simulink model "constraints_comparison_A_4D_v2"  (R2017b)
settings: Solver=ode4  StartTime=0.0  StopTime=10  FixedStep=0.0001  RelTol=1e-3  EnableMultiTasking=on
InitFcn:
  | clear
  | clc
values from neighbouring files (symbols this model uses):
  dail = aircraft_response.Data(:,9)    [dutch_roll_responses_test_plot.m]    (also in short_period_phugoid_responses_test.m)
  dele = aircraft_response.Data(:,10)    [dutch_roll_responses_test_plot.m]    (also in short_period_phugoid_responses_test.m)
  drud = aircraft_response.Data(:,11)    [dutch_roll_responses_test_plot.m]    (also in short_period_phugoid_responses_test.m)
undefined symbols (not defined in the file or in its folder): acm_aero_model, acm_T_N, breakpoints1, Cm0, Cmde, Cmq, de, Fr_mp_1, Fr_mp_2, Fr_rp_1, Fr_rp_2, ini_acm_de_deg, ini_acm_p_deg_per_s, ini_acm_phi_deg, ini_acm_psi_deg, ini_acm_q_deg_per_s, ini_acm_r_deg_per_s, ini_acm_theta_deg, ini_cmp_de_deg, ini_rig_p_deg_per_s, ini_rig_phi_deg, ini_rig_psi_deg, ini_rig_q_deg_per_s, ini_rig_r_deg_per_s, ini_rig_theta_deg, K1_svo_acm, K1_svo_cmp, K2_svo_acm, K2_svo_cmp, La, Ma, max_defl_sat_acm, max_defl_sat_cmp, max_rate_sat, max_rate_sat_acm, max_rate_sat_cmp, Na, sigbuilder_block, simstop, windspeed, Xa, Ya, Za
libraries: aerolibconvert2 x117, simulink x35, sharedtransform x19, vrlib x2
(part 3 of 5)

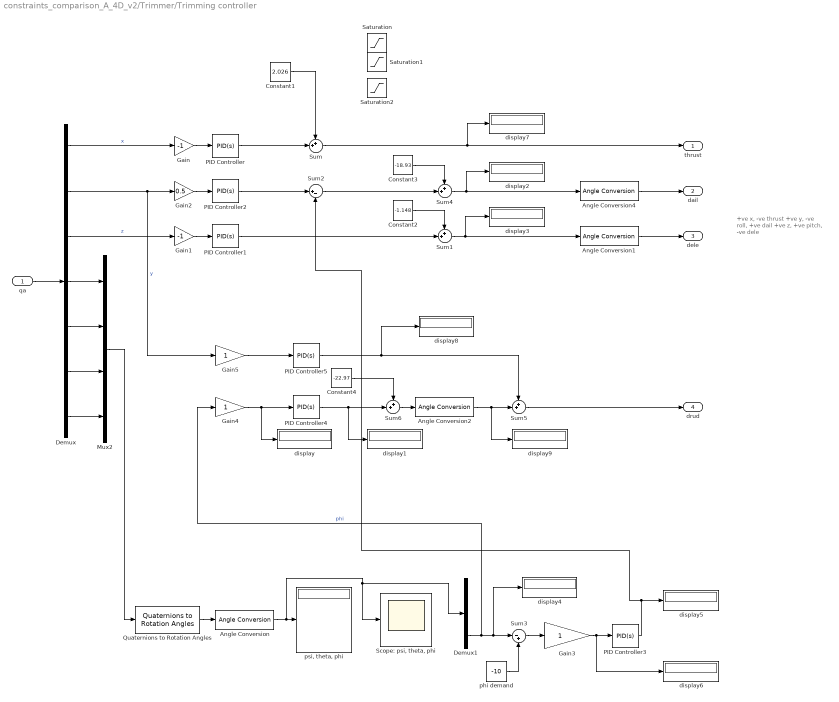
== system constraints_comparison_A_4D_v2/Trimmer/Trimming controller ==
  note: +ve x, -ve thrust
      |
      | +ve y, -ve roll, +ve dail
      |
      | +ve z, +ve pitch, -ve dele
  qa : Inport
  Angle Conversion : aerolibconvert2/Angle Conversion  IU=rad  OU=deg
  Angle Conversion1 : aerolibconvert2/Angle Conversion  IU=deg  OU=rad
  Angle Conversion2 : aerolibconvert2/Angle Conversion  IU=deg  OU=rad
  Angle Conversion4 : aerolibconvert2/Angle Conversion  IU=deg  OU=rad
  Constant1 : Constant  Value=2.026
  Constant2 : Constant  Value=-1.148
  Constant3 : Constant  Value=-18.93
  Constant4 : Constant  Value=-22.97
  Demux : Demux  Outputs=7
  Demux1 : Demux  Outputs=3
  Gain : Gain  Gain=-1
  Gain1 : Gain  Gain=-1
  Gain2 : Gain  Gain=0.5
  Gain3 : Gain
  Gain4 : Gain
  Gain5 : Gain
  Mux2 : Mux
  PID Controller : simulink/Continuous/PID Controller  Controller=PID  TimeDomain=Continuous-time  SampleTime=-1  IntegratorMethod=Forward Euler  FilterMethod=Forward Euler  Form=Parallel  UseFilter=on  ControllerParametersSource=internal  P=2  I=0.5  D=1  N=100  InitialConditionSource=internal  InitialConditionForIntegrator=0  InitialConditionForFilter=0  ExternalReset=none  LimitOutput=off  UpperSaturationLimit=inf  LowerSaturationLimit=-inf  LinearizeAsGain=on  AntiWindupMode=none  Kb=1  TrackingMode=off  Kt=1  PParamMin=[]  PParamMax=[]  IParamMin=[]  IParamMax=[]  DParamMin=[]  DParamMax=[]  NParamMin=[]  NParamMax=[]  KbParamMin=[]  KbParamMax=[]  KtParamMin=[]  KtParamMax=[]  POutMin=[]  POutMax=[]  IOutMin=[]  IOutMax=[]  DOutMin=[]  DOutMax=[]  NOutMin=[]  NOutMax=[]  KbOutMin=[]  KbOutMax=[]  KtOutMin=[]  KtOutMax=[]  IntegratorOutMin=[]  IntegratorOutMax=[]  FilterOutMin=[]  FilterOutMax=[]  SumOutMin=[]  SumOutMax=[]  SumI1OutMin=[]  SumI1OutMax=[]  SumI2OutMin=[]  SumI2OutMax=[]  SumI3OutMin=[]  SumI3OutMax=[]  SumDOutMin=[]  SumDOutMax=[]  SaturationOutMin=[]  SaturationOutMax=[]  IntegratorContinuousStateAttributes=''  IntegratorStateMustResolveToSignalObject=off  IntegratorRTWStateStorageClass=Auto  FilterContinuousStateAttributes=''  FilterStateMustResolveToSignalObject=off  FilterRTWStateStorageClass=Auto  DifferentiatorICPrevScaledInput=0  DifferentiatorOutMin=[]  DifferentiatorOutMax=[]  InitialConditionSetting=State (most efficient)  FilterDiffOutCoefMin=[]  FilterDiffOutCoefMax=[]  SumDenOutMin=[]  SumDenOutMax=[]  SumNumOutMin=[]  SumNumOutMax=[]  ReciprocalOutMin=[]  ReciprocalOutMax=[]  DivideOutMin=[]  DivideOutMax=[]  TunerSelectOption=Transfer Function Based (PID Tuner App)
  PID Controller1 : simulink/Continuous/PID Controller  Controller=PID  TimeDomain=Continuous-time  SampleTime=-1  IntegratorMethod=Forward Euler  FilterMethod=Forward Euler  Form=Parallel  UseFilter=on  ControllerParametersSource=internal  P=2  I=0.5  D=1  N=100  InitialConditionSource=internal  InitialConditionForIntegrator=0  InitialConditionForFilter=0  ExternalReset=none  LimitOutput=off  UpperSaturationLimit=inf  LowerSaturationLimit=-inf  LinearizeAsGain=on  AntiWindupMode=none  Kb=1  TrackingMode=off  Kt=1  PParamMin=[]  PParamMax=[]  IParamMin=[]  IParamMax=[]  DParamMin=[]  DParamMax=[]  NParamMin=[]  NParamMax=[]  KbParamMin=[]  KbParamMax=[]  KtParamMin=[]  KtParamMax=[]  POutMin=[]  POutMax=[]  IOutMin=[]  IOutMax=[]  DOutMin=[]  DOutMax=[]  NOutMin=[]  NOutMax=[]  KbOutMin=[]  KbOutMax=[]  KtOutMin=[]  KtOutMax=[]  IntegratorOutMin=[]  IntegratorOutMax=[]  FilterOutMin=[]  FilterOutMax=[]  SumOutMin=[]  SumOutMax=[]  SumI1OutMin=[]  SumI1OutMax=[]  SumI2OutMin=[]  SumI2OutMax=[]  SumI3OutMin=[]  SumI3OutMax=[]  SumDOutMin=[]  SumDOutMax=[]  SaturationOutMin=[]  SaturationOutMax=[]  IntegratorContinuousStateAttributes=''  IntegratorStateMustResolveToSignalObject=off  IntegratorRTWStateStorageClass=Auto  FilterContinuousStateAttributes=''  FilterStateMustResolveToSignalObject=off  FilterRTWStateStorageClass=Auto  DifferentiatorICPrevScaledInput=0  DifferentiatorOutMin=[]  DifferentiatorOutMax=[]  InitialConditionSetting=State (most efficient)  FilterDiffOutCoefMin=[]  FilterDiffOutCoefMax=[]  SumDenOutMin=[]  SumDenOutMax=[]  SumNumOutMin=[]  SumNumOutMax=[]  ReciprocalOutMin=[]  ReciprocalOutMax=[]  DivideOutMin=[]  DivideOutMax=[]  TunerSelectOption=Transfer Function Based (PID Tuner App)
  PID Controller2 : simulink/Continuous/PID Controller  Controller=PID  TimeDomain=Continuous-time  SampleTime=-1  IntegratorMethod=Forward Euler  FilterMethod=Forward Euler  Form=Parallel  UseFilter=on  ControllerParametersSource=internal  P=0.1  I=0.1  D=0.5  N=100  InitialConditionSource=internal  InitialConditionForIntegrator=0  InitialConditionForFilter=0  ExternalReset=none  LimitOutput=off  UpperSaturationLimit=inf  LowerSaturationLimit=-inf  LinearizeAsGain=on  AntiWindupMode=none  Kb=1  TrackingMode=off  Kt=1  PParamMin=[]  PParamMax=[]  IParamMin=[]  IParamMax=[]  DParamMin=[]  DParamMax=[]  NParamMin=[]  NParamMax=[]  KbParamMin=[]  KbParamMax=[]  KtParamMin=[]  KtParamMax=[]  POutMin=[]  POutMax=[]  IOutMin=[]  IOutMax=[]  DOutMin=[]  DOutMax=[]  NOutMin=[]  NOutMax=[]  KbOutMin=[]  KbOutMax=[]  KtOutMin=[]  KtOutMax=[]  IntegratorOutMin=[]  IntegratorOutMax=[]  FilterOutMin=[]  FilterOutMax=[]  SumOutMin=[]  SumOutMax=[]  SumI1OutMin=[]  SumI1OutMax=[]  SumI2OutMin=[]  SumI2OutMax=[]  SumI3OutMin=[]  SumI3OutMax=[]  SumDOutMin=[]  SumDOutMax=[]  SaturationOutMin=[]  SaturationOutMax=[]  IntegratorContinuousStateAttributes=''  IntegratorStateMustResolveToSignalObject=off  IntegratorRTWStateStorageClass=Auto  FilterContinuousStateAttributes=''  FilterStateMustResolveToSignalObject=off  FilterRTWStateStorageClass=Auto  DifferentiatorICPrevScaledInput=0  DifferentiatorOutMin=[]  DifferentiatorOutMax=[]  InitialConditionSetting=State (most efficient)  FilterDiffOutCoefMin=[]  FilterDiffOutCoefMax=[]  SumDenOutMin=[]  SumDenOutMax=[]  SumNumOutMin=[]  SumNumOutMax=[]  ReciprocalOutMin=[]  ReciprocalOutMax=[]  DivideOutMin=[]  DivideOutMax=[]  TunerSelectOption=Transfer Function Based (PID Tuner App)
  PID Controller3 : simulink/Continuous/PID Controller  Controller=PID  TimeDomain=Continuous-time  SampleTime=-1  IntegratorMethod=Forward Euler  FilterMethod=Forward Euler  Form=Parallel  UseFilter=on  ControllerParametersSource=internal  P=5  I=0.5  D=2  N=100  InitialConditionSource=internal  InitialConditionForIntegrator=0  InitialConditionForFilter=0  ExternalReset=none  LimitOutput=off  UpperSaturationLimit=inf  LowerSaturationLimit=-inf  LinearizeAsGain=on  AntiWindupMode=none  Kb=1  TrackingMode=off  Kt=1  PParamMin=[]  PParamMax=[]  IParamMin=[]  IParamMax=[]  DParamMin=[]  DParamMax=[]  NParamMin=[]  NParamMax=[]  KbParamMin=[]  KbParamMax=[]  KtParamMin=[]  KtParamMax=[]  POutMin=[]  POutMax=[]  IOutMin=[]  IOutMax=[]  DOutMin=[]  DOutMax=[]  NOutMin=[]  NOutMax=[]  KbOutMin=[]  KbOutMax=[]  KtOutMin=[]  KtOutMax=[]  IntegratorOutMin=[]  IntegratorOutMax=[]  FilterOutMin=[]  FilterOutMax=[]  SumOutMin=[]  SumOutMax=[]  SumI1OutMin=[]  SumI1OutMax=[]  SumI2OutMin=[]  SumI2OutMax=[]  SumI3OutMin=[]  SumI3OutMax=[]  SumDOutMin=[]  SumDOutMax=[]  SaturationOutMin=[]  SaturationOutMax=[]  IntegratorContinuousStateAttributes=''  IntegratorStateMustResolveToSignalObject=off  IntegratorRTWStateStorageClass=Auto  FilterContinuousStateAttributes=''  FilterStateMustResolveToSignalObject=off  FilterRTWStateStorageClass=Auto  DifferentiatorICPrevScaledInput=0  DifferentiatorOutMin=[]  DifferentiatorOutMax=[]  InitialConditionSetting=State (most efficient)  FilterDiffOutCoefMin=[]  FilterDiffOutCoefMax=[]  SumDenOutMin=[]  SumDenOutMax=[]  SumNumOutMin=[]  SumNumOutMax=[]  ReciprocalOutMin=[]  ReciprocalOutMax=[]  DivideOutMin=[]  DivideOutMax=[]  TunerSelectOption=Transfer Function Based (PID Tuner App)
  PID Controller4 : simulink/Continuous/PID Controller  Controller=PID  TimeDomain=Continuous-time  SampleTime=-1  IntegratorMethod=Forward Euler  FilterMethod=Forward Euler  Form=Parallel  UseFilter=on  ControllerParametersSource=internal  P=0.1  I=0  D=0  N=100  InitialConditionSource=internal  InitialConditionForIntegrator=0  InitialConditionForFilter=0  ExternalReset=none  LimitOutput=off  UpperSaturationLimit=inf  LowerSaturationLimit=-inf  LinearizeAsGain=on  AntiWindupMode=none  Kb=1  TrackingMode=off  Kt=1  PParamMin=[]  PParamMax=[]  IParamMin=[]  IParamMax=[]  DParamMin=[]  DParamMax=[]  NParamMin=[]  NParamMax=[]  KbParamMin=[]  KbParamMax=[]  KtParamMin=[]  KtParamMax=[]  POutMin=[]  POutMax=[]  IOutMin=[]  IOutMax=[]  DOutMin=[]  DOutMax=[]  NOutMin=[]  NOutMax=[]  KbOutMin=[]  KbOutMax=[]  KtOutMin=[]  KtOutMax=[]  IntegratorOutMin=[]  IntegratorOutMax=[]  FilterOutMin=[]  FilterOutMax=[]  SumOutMin=[]  SumOutMax=[]  SumI1OutMin=[]  SumI1OutMax=[]  SumI2OutMin=[]  SumI2OutMax=[]  SumI3OutMin=[]  SumI3OutMax=[]  SumDOutMin=[]  SumDOutMax=[]  SaturationOutMin=[]  SaturationOutMax=[]  IntegratorContinuousStateAttributes=''  IntegratorStateMustResolveToSignalObject=off  IntegratorRTWStateStorageClass=Auto  FilterContinuousStateAttributes=''  FilterStateMustResolveToSignalObject=off  FilterRTWStateStorageClass=Auto  DifferentiatorICPrevScaledInput=0  DifferentiatorOutMin=[]  DifferentiatorOutMax=[]  InitialConditionSetting=State (most efficient)  FilterDiffOutCoefMin=[]  FilterDiffOutCoefMax=[]  SumDenOutMin=[]  SumDenOutMax=[]  SumNumOutMin=[]  SumNumOutMax=[]  ReciprocalOutMin=[]  ReciprocalOutMax=[]  DivideOutMin=[]  DivideOutMax=[]  TunerSelectOption=Transfer Function Based (PID Tuner App)
  PID Controller5 : simulink/Continuous/PID Controller  Controller=PID  TimeDomain=Continuous-time  SampleTime=-1  IntegratorMethod=Forward Euler  FilterMethod=Forward Euler  Form=Parallel  UseFilter=on  ControllerParametersSource=internal  P=1.0  I=0.3  D=0.3  N=100  InitialConditionSource=internal  InitialConditionForIntegrator=0  InitialConditionForFilter=0  ExternalReset=none  LimitOutput=off  UpperSaturationLimit=inf  LowerSaturationLimit=-inf  LinearizeAsGain=on  AntiWindupMode=none  Kb=1  TrackingMode=off  Kt=1  PParamMin=[]  PParamMax=[]  IParamMin=[]  IParamMax=[]  DParamMin=[]  DParamMax=[]  NParamMin=[]  NParamMax=[]  KbParamMin=[]  KbParamMax=[]  KtParamMin=[]  KtParamMax=[]  POutMin=[]  POutMax=[]  IOutMin=[]  IOutMax=[]  DOutMin=[]  DOutMax=[]  NOutMin=[]  NOutMax=[]  KbOutMin=[]  KbOutMax=[]  KtOutMin=[]  KtOutMax=[]  IntegratorOutMin=[]  IntegratorOutMax=[]  FilterOutMin=[]  FilterOutMax=[]  SumOutMin=[]  SumOutMax=[]  SumI1OutMin=[]  SumI1OutMax=[]  SumI2OutMin=[]  SumI2OutMax=[]  SumI3OutMin=[]  SumI3OutMax=[]  SumDOutMin=[]  SumDOutMax=[]  SaturationOutMin=[]  SaturationOutMax=[]  IntegratorContinuousStateAttributes=''  IntegratorStateMustResolveToSignalObject=off  IntegratorRTWStateStorageClass=Auto  FilterContinuousStateAttributes=''  FilterStateMustResolveToSignalObject=off  FilterRTWStateStorageClass=Auto  DifferentiatorICPrevScaledInput=0  DifferentiatorOutMin=[]  DifferentiatorOutMax=[]  InitialConditionSetting=State (most efficient)  FilterDiffOutCoefMin=[]  FilterDiffOutCoefMax=[]  SumDenOutMin=[]  SumDenOutMax=[]  SumNumOutMin=[]  SumNumOutMax=[]  ReciprocalOutMin=[]  ReciprocalOutMax=[]  DivideOutMin=[]  DivideOutMax=[]  TunerSelectOption=Transfer Function Based (PID Tuner App)
  Quaternions to Rotation Angles : sharedtransform/Quaternions to Rotation Angles  rotationOrder=ZYX
      settings: SourceProductBaseCode=AE
  Saturation : Saturate  UpperLimit=30*pi/180  LowerLimit=-30*pi/180
  Saturation1 : Saturate  UpperLimit=30*pi/180  LowerLimit=-30*pi/180
  Saturation2 : Saturate  UpperLimit=20*pi/180  LowerLimit=-20*pi/180
  "Scope: psi, theta, phi" : Scope
  Sum{,1,4..6} (5 alike) : Sum  Inputs=++|
  Sum2 : Sum  Inputs=|+-
  Sum3 : Sum  Inputs=|-+
  display{,1..9} (10 alike) : Display
  phi demand : Constant  Value=-10
  "psi, theta, phi" : Display
  thrust : Outport
  dail : Outport  Port=2
  dele : Outport  Port=3
  drud : Outport  Port=4
  wires:
  qa/1 -> Demux/1
  Demux/4 -> Mux2/1
  Demux/5 -> Mux2/2
  Demux/6 -> Mux2/3
  Demux/7 -> Mux2/4
  Demux/1 -> Gain/1  "x"
  Demux/2 -> Gain5/1, Gain2/1  "y"
  Demux/3 -> Gain1/1  "z"
  Gain/1 -> PID Controller/1
  Gain1/1 -> PID Controller1/1
  Gain2/1 -> PID Controller2/1
  PID Controller1/1 -> Sum1/2
  Sum/1 -> display7/1, thrust/1
  PID Controller/1 -> Sum/2
  Constant1/1 -> Sum/1
  Sum4/1 -> Angle Conversion4/1, display2/1
  Constant2/1 -> Sum1/1
  Sum1/1 -> Angle Conversion1/1, display3/1
  Angle Conversion4/1 -> dail/1
  Angle Conversion1/1 -> dele/1
  Angle Conversion2/1 -> display9/1, Sum5/2
  Mux2/1 -> Quaternions to Rotation Angles/1
  Quaternions to Rotation Angles/1 -> Angle Conversion/1
  Angle Conversion/1 -> Demux1/1, "Scope: psi, theta, phi"/1, "psi, theta, phi"/1
  PID Controller2/1 -> Sum2/1
  Gain3/1 -> display6/1, PID Controller3/1
  Demux1/3 -> Gain4/1, display4/1, Sum3/1  "phi"
  PID Controller3/1 -> Sum2/2, display5/1
  Sum3/1 -> Gain3/1
  phi demand/1 -> Sum3/2
  Gain4/1 -> PID Controller4/1, display/1
  PID Controller4/1 -> Sum6/2, display1/1
  Sum5/1 -> drud/1
  Gain5/1 -> PID Controller5/1
  PID Controller5/1 -> display8/1, Sum5/1
  Sum2/1 -> Sum4/2
  Constant3/1 -> Sum4/1
  Sum6/1 -> Angle Conversion2/1
  Constant4/1 -> Sum6/1

== system constraints_comparison_A_4D_v2/Control surface input/1) Short period/Signal Builder ==
  Demux : Demux  Tag=STV Demux  Outputs=1
  FromWs : FromWorkspace  Tag=STV FromWs  VariableName=tuvar  SampleTime=0
      SigBuilderData=|
      | common.afterFinalStr = 'Extrapolate'
      | common.sampleTime = 0
      | dataSet.timeRange = [0 100]
      | dataSet.name = 'Group 1'
      | sbobj.Groups.Name = 'Group 1'
      | sbobj.Groups.Signals.Name = 'Signal 1'
      | sbobj.Groups.Signals.XData = [0 2 2 2.25 2.25 100]
      | sbobj.Groups.Signals.YData = [0 0 -1 -1 0 0]
      | sbobj.Groups.TimeRange = [0 100]
  Signal 1 : Outport  Tag=STV Outport
  wires:
  Demux/1 -> Signal 1/1
  FromWs/1 -> Demux/1

== system constraints_comparison_A_4D_v2/Control surface input/2) Phugoid/Signal Builder ==
  Demux : Demux  Tag=STV Demux  Outputs=1
  FromWs : FromWorkspace  Tag=STV FromWs  VariableName=tuvar  SampleTime=0
      SigBuilderData=|
      | common.afterFinalStr = 'Extrapolate'
      | common.sampleTime = 0
      | dataSet.timeRange = [0 100]
      | dataSet.name = 'Group 1'
      | sbobj.Groups.Name = 'Group 1'
      | sbobj.Groups.Signals.Name = 'Signal 1'
      | sbobj.Groups.Signals.XData = [0 2 2 2.25 2.25 2.5 2.5 100]
      | sbobj.Groups.Signals.YData = [0 0 -1 -1 1 1 0 0]
      | sbobj.Groups.TimeRange = [0 100]
  Signal 1 : Outport  Tag=STV Outport
  wires:
  Demux/1 -> Signal 1/1
  FromWs/1 -> Demux/1

== system constraints_comparison_A_4D_v2/Control surface input/3) Roll subsidence/Signal Builder ==
  Demux : Demux  Tag=STV Demux  Outputs=1
  FromWs : FromWorkspace  Tag=STV FromWs  VariableName=tuvar  SampleTime=0
      SigBuilderData=|
      | common.afterFinalStr = 'Extrapolate'
      | common.sampleTime = 0
      | dataSet.timeRange = [0 100]
      | dataSet.name = 'Group 1'
      | sbobj.Groups.Name = 'Group 1'
      | sbobj.Groups.Signals.Name = 'Signal 1'
      | sbobj.Groups.Signals.XData = [0 1 1 1.5 1.5 100]
      | sbobj.Groups.Signals.YData = [0 0 -0.5 -0.5 0 0]
      | sbobj.Groups.TimeRange = [0 100]
  Signal 1 : Outport  Tag=STV Outport
  wires:
  Demux/1 -> Signal 1/1
  FromWs/1 -> Demux/1

== system constraints_comparison_A_4D_v2/Control surface input/3) Roll subsidence/Signal Builder1 ==
  Demux : Demux  Tag=STV Demux  Outputs=1
  FromWs : FromWorkspace  Tag=STV FromWs  VariableName=tuvar  SampleTime=0
      SigBuilderData=|
      | common.afterFinalStr = 'Extrapolate'
      | common.sampleTime = 0
      | dataSet.timeRange = [0 100]
      | dataSet.name = 'Group 1'
      | sbobj.Groups.Name = 'Group 1'
      | sbobj.Groups.Signals.Name = 'Signal 1'
      | sbobj.Groups.Signals.XData = [0 1 1 1.67 1.67 100]
      | sbobj.Groups.Signals.YData = [0 0 -0.67 -0.67 0 0]
      | sbobj.Groups.TimeRange = [0 100]
  Signal 1 : Outport  Tag=STV Outport
  wires:
  FromWs/1 -> Demux/1
  Demux/1 -> Signal 1/1

== system constraints_comparison_A_4D_v2/Control surface input/4) Spiral/Signal Builder1 ==
  Demux : Demux  Tag=STV Demux  Outputs=1
  FromWs : FromWorkspace  Tag=STV FromWs  VariableName=tuvar  SampleTime=0
      SigBuilderData=|
      | common.afterFinalStr = 'Extrapolate'
      | common.sampleTime = 0
      | dataSet.timeRange = [0 100]
      | dataSet.name = 'Group 1'
      | sbobj.Groups.Name = 'Group 1'
      | sbobj.Groups.Signals.Name = 'Signal 1'
      | sbobj.Groups.Signals.XData = [0 2 2 100]
      | sbobj.Groups.Signals.YData = [0 0 -1 -1]
      | sbobj.Groups.TimeRange = [0 100]
  Signal 1 : Outport  Tag=STV Outport
  wires:
  Demux/1 -> Signal 1/1
  FromWs/1 -> Demux/1

== system constraints_comparison_A_4D_v2/Control surface input/5) Dutch roll/Signal Builder ==
  Demux : Demux  Tag=STV Demux  Outputs=1
  FromWs : FromWorkspace  Tag=STV FromWs  VariableName=tuvar  SampleTime=0
      SigBuilderData=|
      | common.afterFinalStr = 'Extrapolate'
      | common.sampleTime = 0
      | dataSet.timeRange = [0 100]
      | dataSet.name = 'Group 1'
      | sbobj.Groups.Name = 'Group 1'
      | sbobj.Groups.Signals.Name = 'Signal 1'
      | sbobj.Groups.Signals.XData = [0 2 2 2.8747 2.8747 3.7494 3.7494 100]
      | sbobj.Groups.Signals.YData = [0 0 -1 -1 1 1 0 0]
      | sbobj.Groups.TimeRange = [0 100]
  Signal 1 : Outport  Tag=STV Outport
  wires:
  Demux/1 -> Signal 1/1
  FromWs/1 -> Demux/1

== system constraints_comparison_A_4D_v2/Control surface input/5) Dutch roll/Signal Builder1 ==
  Demux : Demux  Tag=STV Demux  Outputs=1
  FromWs : FromWorkspace  Tag=STV FromWs  VariableName=tuvar  SampleTime=0
      SigBuilderData=|
      | common.afterFinalStr = 'Extrapolate'
      | common.sampleTime = 0
      | dataSet.timeRange = [0 100]
      | dataSet.name = 'Group 1'
      | sbobj.Groups.Name = 'Group 1'
      | sbobj.Groups.Signals.Name = 'Signal 1'
      | sbobj.Groups.Signals.XData = [0 2 2 2.2426 2.2426 2.4852 2.4852 100]
      | sbobj.Groups.Signals.YData = [0 0 -1 -1 1 1 0 0]
      | sbobj.Groups.TimeRange = [0 100]
  Signal 1 : Outport  Tag=STV Outport
  wires:
  Demux/1 -> Signal 1/1
  FromWs/1 -> Demux/1

== system constraints_comparison_A_4D_v2/Control surface input/5) Dutch roll/Signal Builder1 old (two dublets) ==
  Demux : Demux  Tag=STV Demux  Outputs=1
  FromWs : FromWorkspace  Tag=STV FromWs  VariableName=tuvar  SampleTime=0
      SigBuilderData=|
      | common.afterFinalStr = 'Extrapolate'
      | common.sampleTime = 0
      | dataSet.timeRange = [0 100]
      | dataSet.name = 'Group 1'
      | sbobj.Groups.Name = 'Group 1'
      | sbobj.Groups.Signals.Name = 'Signal 1'
      | sbobj.Groups.Signals.XData = [0 2 2 2.2426 2.2426 2.4852 2.4852 4.5 4.5 4.7426 4.7426 4.9852 4.9852 100]
      | sbobj.Groups.Signals.YData = [0 0 -1 -1 1 1 0 0 1 1 -1 -1 0 0]
      | sbobj.Groups.TimeRange = [0 100]
  Signal 1 : Outport  Tag=STV Outport
  wires:
  FromWs/1 -> Demux/1
  Demux/1 -> Signal 1/1

== system constraints_comparison_A_4D_v2/Subsystem14/Compensator servo model1/kinematic ==
  note: If position saturation limit is reached, rate integration is reset
  rate_dot : Inport
  Angle Conversion : aerolibconvert2/Angle Conversion  IU=deg  OU=rad
  Compare To Zero : simulink/Logic and Bit Operations/Compare To Zero  relop=>  OutDataTypeStr=boolean  ZeroCross=off
  Compare To Zero1 : simulink/Logic and Bit Operations/Compare To Zero  relop=<  OutDataTypeStr=boolean  ZeroCross=off
  Compare To Zero2 : simulink/Logic and Bit Operations/Compare To Zero  relop=>  OutDataTypeStr=boolean  ZeroCross=off
  Compare To Zero3 : simulink/Logic and Bit Operations/Compare To Zero  relop=<  OutDataTypeStr=boolean  ZeroCross=off
  Logical Operator : Logic  Operator=OR  AllPortsSameDT=off  OutDataTypeStr=boolean
  Logical Operator1 : Logic  AllPortsSameDT=off  OutDataTypeStr=boolean
  Logical Operator2 : Logic  AllPortsSameDT=off  OutDataTypeStr=boolean
  ini_cmp_de_deg : Constant  Value=ini_cmp_de_deg
  pos : Integrator  InitialConditionSource=external  LimitOutput=on  UpperSaturationLimit=max_defl_sat_cmp  LowerSaturationLimit=-max_defl_sat_cmp  ShowSaturationPort=on  ZeroCross=off
  rate : Integrator  ExternalReset=level hold  UpperSaturationLimit=max_rate_sat  LowerSaturationLimit=-max_rate_sat  ZeroCross=off
  de : Outport
  de_dot : Outport  Port=2
  wires:
  Compare To Zero/1 -> Logical Operator1/1
  Logical Operator/1 -> rate/2
  Logical Operator1/1 -> Logical Operator/1
  rate_dot/1 -> rate/1
  pos/1 -> de/1
  rate/1 -> Compare To Zero1/1, Compare To Zero/1, de_dot/1, pos/1
  Compare To Zero2/1 -> Logical Operator1/2
  Logical Operator2/1 -> Logical Operator/2
  Compare To Zero1/1 -> Logical Operator2/1
  Compare To Zero3/1 -> Logical Operator2/2
  pos/2 -> Compare To Zero3/1, Compare To Zero2/1
  ini_cmp_de_deg/1 -> Angle Conversion/1
  Angle Conversion/1 -> pos/2

== system constraints_comparison_A_4D_v2/Subsystem14/Compensator servo model2/kinematic ==
  note: If position saturation limit is reached, rate integration is reset
  rate_dot : Inport
  Angle Conversion : aerolibconvert2/Angle Conversion  IU=deg  OU=rad
  Compare To Zero : simulink/Logic and Bit Operations/Compare To Zero  relop=>  OutDataTypeStr=boolean  ZeroCross=off
  Compare To Zero1 : simulink/Logic and Bit Operations/Compare To Zero  relop=<  OutDataTypeStr=boolean  ZeroCross=off
  Compare To Zero2 : simulink/Logic and Bit Operations/Compare To Zero  relop=>  OutDataTypeStr=boolean  ZeroCross=off
  Compare To Zero3 : simulink/Logic and Bit Operations/Compare To Zero  relop=<  OutDataTypeStr=boolean  ZeroCross=off
  Gain8 : Gain  Gain=-1
  Logical Operator : Logic  Operator=OR  AllPortsSameDT=off  OutDataTypeStr=boolean
  Logical Operator1 : Logic  AllPortsSameDT=off  OutDataTypeStr=boolean
  Logical Operator2 : Logic  AllPortsSameDT=off  OutDataTypeStr=boolean
  ini_cmp_de_deg : Constant  Value=ini_cmp_de_deg
  pos : Integrator  InitialConditionSource=external  LimitOutput=on  UpperSaturationLimit=max_defl_sat_cmp  LowerSaturationLimit=-max_defl_sat_cmp  ShowSaturationPort=on  ZeroCross=off
  rate : Integrator  ExternalReset=level hold  UpperSaturationLimit=max_rate_sat  LowerSaturationLimit=-max_rate_sat  ZeroCross=off
  de : Outport
  de_dot : Outport  Port=2
  wires:
  Angle Conversion/1 -> pos/2
  ini_cmp_de_deg/1 -> Gain8/1
  pos/2 -> Compare To Zero2/1, Compare To Zero3/1
  Compare To Zero3/1 -> Logical Operator2/2
  Compare To Zero1/1 -> Logical Operator2/1
  Logical Operator2/1 -> Logical Operator/2
  Compare To Zero2/1 -> Logical Operator1/2
  rate/1 -> pos/1, de_dot/1, Compare To Zero/1, Compare To Zero1/1
  pos/1 -> de/1
  rate_dot/1 -> rate/1
  Logical Operator1/1 -> Logical Operator/1
  Logical Operator/1 -> rate/2
  Compare To Zero/1 -> Logical Operator1/1
  Gain8/1 -> Angle Conversion/1

== system constraints_comparison_A_4D_v2/Subsystem14/Compensator servo model3/kinematic ==
  note: If position saturation limit is reached, rate integration is reset
  rate_dot : Inport
  Angle Conversion : aerolibconvert2/Angle Conversion  IU=deg  OU=rad
  Compare To Zero : simulink/Logic and Bit Operations/Compare To Zero  relop=>  OutDataTypeStr=boolean  ZeroCross=off
  Compare To Zero1 : simulink/Logic and Bit Operations/Compare To Zero  relop=<  OutDataTypeStr=boolean  ZeroCross=off
  Compare To Zero2 : simulink/Logic and Bit Operations/Compare To Zero  relop=>  OutDataTypeStr=boolean  ZeroCross=off
  Compare To Zero3 : simulink/Logic and Bit Operations/Compare To Zero  relop=<  OutDataTypeStr=boolean  ZeroCross=off
  Gain8 : Gain  Gain=-1
  Logical Operator : Logic  Operator=OR  AllPortsSameDT=off  OutDataTypeStr=boolean
  Logical Operator1 : Logic  AllPortsSameDT=off  OutDataTypeStr=boolean
  Logical Operator2 : Logic  AllPortsSameDT=off  OutDataTypeStr=boolean
  ini_cmp_de_deg : Constant  Value=ini_cmp_de_deg
  pos : Integrator  InitialConditionSource=external  LimitOutput=on  UpperSaturationLimit=max_defl_sat_cmp  LowerSaturationLimit=-max_defl_sat_cmp  ShowSaturationPort=on  ZeroCross=off
  rate : Integrator  ExternalReset=level hold  UpperSaturationLimit=max_rate_sat  LowerSaturationLimit=-max_rate_sat  ZeroCross=off
  de : Outport
  de_dot : Outport  Port=2
  wires:
  Compare To Zero/1 -> Logical Operator1/1
  Logical Operator/1 -> rate/2
  Logical Operator1/1 -> Logical Operator/1
  rate_dot/1 -> rate/1
  pos/1 -> de/1
  rate/1 -> Compare To Zero1/1, Compare To Zero/1, de_dot/1, pos/1
  Compare To Zero2/1 -> Logical Operator1/2
  Logical Operator2/1 -> Logical Operator/2
  Compare To Zero1/1 -> Logical Operator2/1
  Compare To Zero3/1 -> Logical Operator2/2
  pos/2 -> Compare To Zero3/1, Compare To Zero2/1
  ini_cmp_de_deg/1 -> Gain8/1
  Angle Conversion/1 -> pos/2
  Gain8/1 -> Angle Conversion/1

== system constraints_comparison_A_4D_v2/Subsystem14/Compensator servo model4/kinematic ==
  note: If position saturation limit is reached, rate integration is reset
  rate_dot : Inport
  Angle Conversion : aerolibconvert2/Angle Conversion  IU=deg  OU=rad
  Compare To Zero : simulink/Logic and Bit Operations/Compare To Zero  relop=>  OutDataTypeStr=boolean  ZeroCross=off
  Compare To Zero1 : simulink/Logic and Bit Operations/Compare To Zero  relop=<  OutDataTypeStr=boolean  ZeroCross=off
  Compare To Zero2 : simulink/Logic and Bit Operations/Compare To Zero  relop=>  OutDataTypeStr=boolean  ZeroCross=off
  Compare To Zero3 : simulink/Logic and Bit Operations/Compare To Zero  relop=<  OutDataTypeStr=boolean  ZeroCross=off
  Logical Operator : Logic  Operator=OR  AllPortsSameDT=off  OutDataTypeStr=boolean
  Logical Operator1 : Logic  AllPortsSameDT=off  OutDataTypeStr=boolean
  Logical Operator2 : Logic  AllPortsSameDT=off  OutDataTypeStr=boolean
  ini_cmp_de_deg : Constant  Value=ini_cmp_de_deg
  pos : Integrator  InitialConditionSource=external  LimitOutput=on  UpperSaturationLimit=max_defl_sat_cmp  LowerSaturationLimit=-max_defl_sat_cmp  ShowSaturationPort=on  ZeroCross=off
  rate : Integrator  ExternalReset=level hold  UpperSaturationLimit=max_rate_sat  LowerSaturationLimit=-max_rate_sat  ZeroCross=off
  de : Outport
  de_dot : Outport  Port=2
  wires:
  Angle Conversion/1 -> pos/2
  ini_cmp_de_deg/1 -> Angle Conversion/1
  pos/2 -> Compare To Zero2/1, Compare To Zero3/1
  Compare To Zero3/1 -> Logical Operator2/2
  Compare To Zero1/1 -> Logical Operator2/1
  Logical Operator2/1 -> Logical Operator/2
  Compare To Zero2/1 -> Logical Operator1/2
  rate/1 -> pos/1, de_dot/1, Compare To Zero/1, Compare To Zero1/1
  pos/1 -> de/1
  rate_dot/1 -> rate/1
  Logical Operator1/1 -> Logical Operator/1
  Logical Operator/1 -> rate/2
  Compare To Zero/1 -> Logical Operator1/1

== system constraints_comparison_A_4D_v2/Subsystem14/Hawk servo model/kinematic ==
  note: If position saturation limit is reached, rate integration is reset
  rate_dot : Inport
  Angle Conversion : aerolibconvert2/Angle Conversion  IU=deg  OU=rad
  Compare To Zero : simulink/Logic and Bit Operations/Compare To Zero  relop=>  OutDataTypeStr=boolean  ZeroCross=off
  Compare To Zero1 : simulink/Logic and Bit Operations/Compare To Zero  relop=<  OutDataTypeStr=boolean  ZeroCross=off
  Compare To Zero2 : simulink/Logic and Bit Operations/Compare To Zero  relop=>  OutDataTypeStr=boolean  ZeroCross=off
  Compare To Zero3 : simulink/Logic and Bit Operations/Compare To Zero  relop=<  OutDataTypeStr=boolean  ZeroCross=off
  Linear aero model trim (higher accuracy) : Constant  Value=1.1658924813874*pi/180
  Linear aero model trim (higher accuracy)1 : Constant  Value=4.4011
  Logical Operator : Logic  Operator=OR  AllPortsSameDT=off  OutDataTypeStr=boolean
  Logical Operator1 : Logic  AllPortsSameDT=off  OutDataTypeStr=boolean
  Logical Operator2 : Logic  AllPortsSameDT=off  OutDataTypeStr=boolean
  ini_acm_de_deg : Constant  Value=ini_acm_de_deg
  pos : Integrator  InitialConditionSource=external  LimitOutput=on  UpperSaturationLimit=max_defl_sat_acm  LowerSaturationLimit=-max_defl_sat_acm  ShowSaturationPort=on  ZeroCross=off
  rate : Integrator  ExternalReset=level hold  UpperSaturationLimit=max_rate_sat  LowerSaturationLimit=-max_rate_sat  ZeroCross=off
  de : Outport
  de_dot : Outport  Port=2
  wires:
  Compare To Zero/1 -> Logical Operator1/1
  Logical Operator/1 -> rate/2
  Logical Operator1/1 -> Logical Operator/1
  rate_dot/1 -> rate/1
  pos/1 -> de/1
  rate/1 -> Compare To Zero1/1, Compare To Zero/1, de_dot/1, pos/1
  Compare To Zero2/1 -> Logical Operator1/2
  Logical Operator2/1 -> Logical Operator/2
  Compare To Zero1/1 -> Logical Operator2/1
  Compare To Zero3/1 -> Logical Operator2/2
  pos/2 -> Compare To Zero3/1, Compare To Zero2/1
  Linear aero model trim (higher accuracy)/1 -> ?
  ini_acm_de_deg/1 -> Angle Conversion/1
  Angle Conversion/1 -> pos/2

== matlab function constraints_comparison_A_4D_v2/Subsystem14/MATLAB Function1 ==
  data: A2 input; A22 output
function A22 = fcn(A2)

A22 = [ A2(1,1)
        A2(2,1)
        A2(3,1)
        A2(1,2)
        A2(2,2)
        A2(3,2)
        A2(1,3)
        A2(2,3)
        A2(3,3) ];
